simulink model "RobotControl"  (R2016a)
settings: Solver=FixedStepDiscrete  StartTime=0.0  StopTime=16  FixedStep=0.005  RelTol=1e-3
undefined symbols (not defined in the file or in its folder): CAL_EAST, CAL_NORTH, CAL_SOUTH, CAL_thetaGain, CAL_WEST, ENU_END, ENU_FORWARD, ENU_GTSP, ENU_LEFT_BUSY_RIGHT_BUSY, ENU_LEFT_BUSY_RIGHT_CLEANED, ENU_LEFT_BUSY_RIGHT_EMPTY, ENU_LEFT_CLEANED_RIGHT_BUSY, ENU_LEFT_CLEANED_RIGHT_CLEANED, ENU_LEFT_CLEANED_RIGHT_EMPTY, ENU_LEFT_EMPTY_RIGHT_BUSY, ENU_LEFT_EMPTY_RIGHT_CLEANED, ENU_LEFT_EMPTY_RIGHT_EMPTY, ENU_MOVE_TURN_LEFT, ENU_MOVE_TURN_RIGHT, ENU_MOVE_U_TURN, ENU_MOVE_U_TURN_LEFT, ENU_MOVE_U_TURN_RIGHT, ENU_STOP, ENU_ZIGZAG, ROTH, Routines
libraries: COMH x1, MOVH x1, SCAN x1, MOTH x1
settings Model: Creator=oelkawok  LastModifiedBy=oelkawok
settings DataIOCC: SaveOutput=off  SaveTime=off
settings DebuggingCC: AlgebraicLoopMsg=error  UnnecessaryDatatypeConvMsg=warning  SFcnCompatibilityMsg=warning

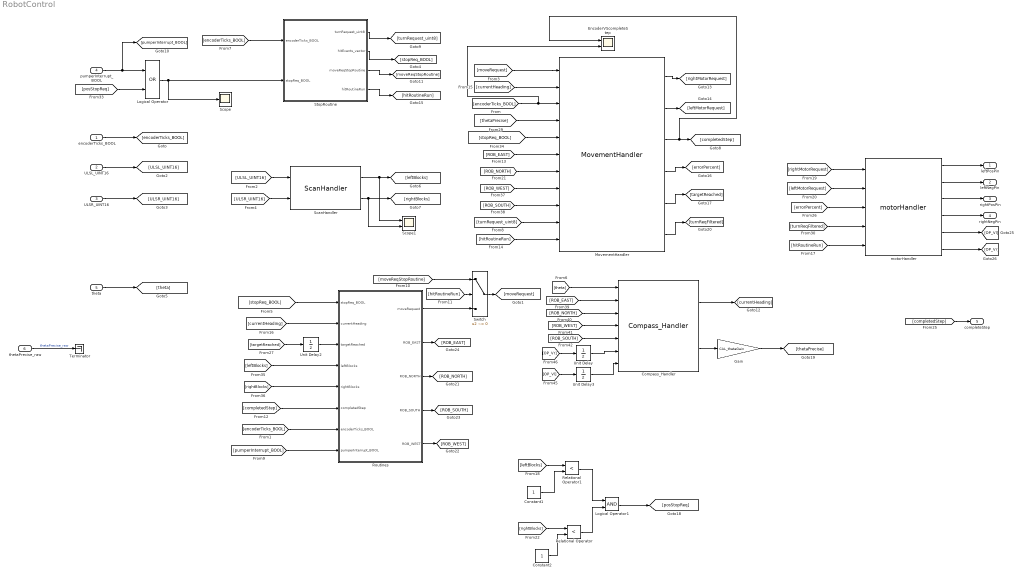
== system RobotControl ==
  encoderTicks_BOOL : Inport  OutDataTypeStr=boolean  PortDimensions=1
  ULSL_UINT16 : Inport  Port=2  PortDimensions=1
  ULSR_UINT16 : Inport  Port=3  PortDimensions=1
  pumperInterrupt_BOOL : Inport  Port=4  OutDataTypeStr=boolean  PortDimensions=1
  theta : Inport  Port=5  OutDataTypeStr=int16  PortDimensions=1
  thetaPrecise_raw : Inport  Port=6  OutDataTypeStr=uint16  PortDimensions=1
  Compass_Handler : COMH/Compass_Handler
  Constant1 : Constant
  Constant2 : Constant
  EncoderVScompleteStep : Scope  NumInputPorts=2
  Gain : Gain  Gain=CAL_thetaGain
  Logical Operator : Logic  Operator=OR  AllPortsSameDT=off  OutDataTypeStr=boolean
  Logical Operator1 : Logic  AllPortsSameDT=off  OutDataTypeStr=boolean
  MovementHandler : MOVH/MovementHandler
  Relational Operator : RelationalOperator  Operator=<  OutDataTypeStr=boolean
  Relational Operator1 : RelationalOperator  Operator=<  OutDataTypeStr=boolean
  Routines : Subsystem  AncestorBlock=ROTH/Routines
  ScanHandler : SCAN/ScanHandler
  Scope : Scope
  Scope1 : Scope  NumInputPorts=2
  StopRoutine : Subsystem
  Switch : Switch  Criteria=u2 ~= 0
  Terminator : Terminator
  Unit Delay : UnitDelay  SampleTime=-1
  Unit Delay2 : UnitDelay  SampleTime=-1
  Unit Delay3 : UnitDelay  SampleTime=-1
  motorHandler : MOTH/motorHandler
  leftPosPin : Outport  OutDataTypeStr=uint8  PortDimensions=1
  leftNegPin : Outport  Port=2  OutDataTypeStr=uint8  PortDimensions=1
  rightPosPin : Outport  Port=3  OutDataTypeStr=uint8  PortDimensions=1
  rightNegPin : Outport  Port=4  OutDataTypeStr=uint8  PortDimensions=1
  completeStep : Outport  Port=5  PortDimensions=1
  wires:
  [moveRequest] -> MovementHandler/1
  [encoderTicks_BOOL] -> EncoderVScompleteStep/2, MovementHandler/3
  encoderTicks_BOOL/1 -> [encoderTicks_BOOL]
  ULSL_UINT16/1 -> [ULSL_UINT16]
  [ULSL_UINT16] -> ScanHandler/1
  ULSR_UINT16/1 -> [ULSR_UINT16]
  [ULSR_UINT16] -> ScanHandler/2
  [theta] -> Compass_Handler/1
  ScanHandler/1 -> Scope1/1, [leftBlocks]
  ScanHandler/2 -> Scope1/2, [rightBlocks]
  MovementHandler/3 -> EncoderVScompleteStep/1, [completedStep]
  Compass_Handler/1 -> [currentHeading]
  [currentHeading] -> MovementHandler/2
  [rightMotorRequest] -> motorHandler/1
  [leftMotorRequest] -> motorHandler/2
  MovementHandler/2 -> [leftMotorRequest]
  MovementHandler/1 -> [rightMotorRequest]
  motorHandler/4 -> rightNegPin/1
  motorHandler/2 -> leftNegPin/1
  motorHandler/3 -> rightPosPin/1
  motorHandler/1 -> leftPosPin/1
  [completedStep] -> completeStep/1
  [errorPercent] -> motorHandler/3
  MovementHandler/4 -> [errorPercent]
  MovementHandler/5 -> [targetReached]
  [targetReached] -> Unit Delay2/1
  theta/1 -> [theta]
  [thetaPrecise] -> MovementHandler/4
  MovementHandler/6 -> [turnReqFiltered]
  [turnReqFiltered] -> motorHandler/4
  pumperInterrupt_BOOL/1 -> [pumperInterrupt_BOOL], Logical Operator/1
  [posStopReq] -> Logical Operator/2
  Logical Operator/1 -> Scope/1, StopRoutine/2(stopReq_BOOL)
  [stopReq_BOOL] -> MovementHandler/5
  Unit Delay2/1 -> Routines/3(targetReached)
  [stopReq_BOOL] -> Routines/1(stopReq_BOOL)
  [rightBlocks] -> Routines/5(rightBlocks)
  [leftBlocks] -> Routines/4(leftBlocks)
  [currentHeading] -> Routines/2(currentHeading)
  Logical Operator1/1 -> [posStopReq]
  [completedStep] -> Routines/6(completedStep)
  Routines/3(ROB_NORTH) -> [ROB_NORTH]
  Routines/2(ROB_EAST) -> [ROB_EAST]
  Routines/4(ROB_SOUTH) -> [ROB_SOUTH]
  Routines/5(ROB_WEST) -> [ROB_WEST]
  [ROB_NORTH] -> MovementHandler/7
  [ROB_EAST] -> MovementHandler/6
  [ROB_WEST] -> MovementHandler/8
  [ROB_SOUTH] -> MovementHandler/9
  [ROB_EAST] -> Compass_Handler/2
  [ROB_NORTH] -> Compass_Handler/3
  [ROB_WEST] -> Compass_Handler/4
  [ROB_SOUTH] -> Compass_Handler/5
  motorHandler/5 -> [OP_Vl]
  motorHandler/6 -> [OP_Vr]
  [OP_Vr] -> Unit Delay/1
  [OP_Vl] -> Unit Delay3/1
  Unit Delay/1 -> Compass_Handler/6
  Unit Delay3/1 -> Compass_Handler/7
  Compass_Handler/2 -> Gain/1
  Gain/1 -> [thetaPrecise]
  thetaPrecise_raw/1 -> Terminator/1  "thetaPrecise_raw"
  [encoderTicks_BOOL] -> Routines/7(encoderTicks_BOOL)
  [encoderTicks_BOOL] -> StopRoutine/1(encoderTicks_BOOL)
  StopRoutine/2(hitEvents_vector) -> [stopReq_BOOL]
  StopRoutine/1(turnRequest_uint8) -> [turnRequest_uint8]
  [turnRequest_uint8] -> MovementHandler/10
  [pumperInterrupt_BOOL] -> Routines/8(pumperInterrupt_BOOL)
  StopRoutine/3(moveReqStopRoutine) -> [moveReqStopRoutine]
  Switch/1 -> [moveRequest]
  Routines/1(moveRequest) -> Switch/3
  [moveReqStopRoutine] -> Switch/1
  StopRoutine/4(hitRoutineRun) -> [hitRoutineRun]
  [hitRoutineRun] -> Switch/2
  [hitRoutineRun] -> MovementHandler/11
  [hitRoutineRun] -> motorHandler/5
  [rightBlocks] -> Relational Operator/1
  Constant2/1 -> Relational Operator/2
  [leftBlocks] -> Relational Operator1/1
  Constant1/1 -> Relational Operator1/2
  Relational Operator1/1 -> Logical Operator1/1
  Relational Operator/1 -> Logical Operator1/2

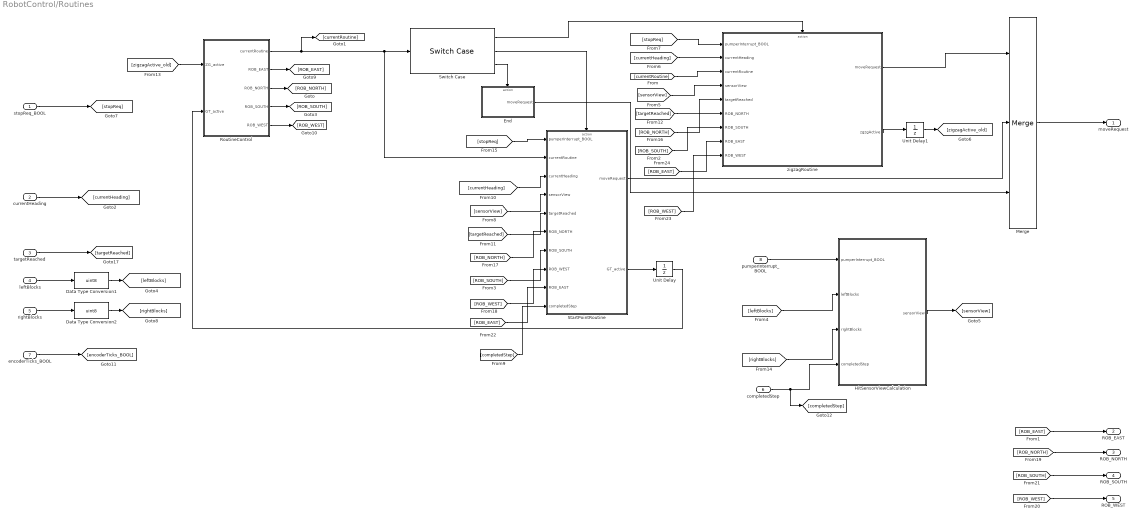
== system RobotControl/Routines ==
  stopReq_BOOL : Inport
  currentHeading : Inport  Port=2
  targetReached : Inport  Port=3
  leftBlocks : Inport  Port=4
  rightBlocks : Inport  Port=5
  completedStep : Inport  Port=6
  encoderTicks_BOOL : Inport  Port=7
  pumperInterrupt_BOOL : Inport  Port=8
  Data Type Conversion1 : DataTypeConversion  OutDataTypeStr=uint8
  Data Type Conversion2 : DataTypeConversion  OutDataTypeStr=uint8
  End : Subsystem  TreatAsAtomicUnit=on
  HitSensorViewCalculation : Subsystem
  Merge : Merge  Inputs=3  InitialOutput=5
      settings: AttributesFormatString=%<InitialOutput>
  RoutineControl : Subsystem
  StartPointRoutine : Subsystem
  Switch Case : SwitchCase  CaseConditions={ENU_ZIGZAG, ENU_GTSP, ENU_END}  ShowDefaultCase=off
      settings: AttributesFormatString=%<CaseConditions>
  Unit Delay : UnitDelay  InitialCondition=true  SampleTime=-1
      settings: AttributesFormatString=%<InitialCondition>
  Unit Delay1 : UnitDelay  InitialCondition=false  SampleTime=-1
      settings: AttributesFormatString=%<InitialCondition>
  zigzagRoutine : Subsystem
  moveRequest : Outport
  ROB_EAST : Outport  Port=2
  ROB_NORTH : Outport  Port=3
  ROB_SOUTH : Outport  Port=4
  ROB_WEST : Outport  Port=5
  wires:
  completedStep/1 -> [completedStep], HitSensorViewCalculation/4(completedStep)
  [leftBlocks] -> HitSensorViewCalculation/2(leftBlocks)
  [rightBlocks] -> HitSensorViewCalculation/3(rightBlocks)
  Data Type Conversion2/1 -> [rightBlocks]
  Data Type Conversion1/1 -> [leftBlocks]
  rightBlocks/1 -> Data Type Conversion2/1
  leftBlocks/1 -> Data Type Conversion1/1
  [zigzagActive_old] -> RoutineControl/1(ZG_active)
  Unit Delay1/1 -> [zigzagActive_old]
  [currentRoutine] -> zigzagRoutine/3(currentRoutine)
  currentHeading/1 -> [currentHeading]
  Unit Delay/1 -> RoutineControl/2(GT_active)
  StartPointRoutine/2(GT_active) -> Unit Delay/1
  Merge/1 -> moveRequest/1
  HitSensorViewCalculation/1(sensorView) -> [sensorView]
  [sensorView] -> zigzagRoutine/4(sensorView)
  [stopReq] -> zigzagRoutine/1(pumperInterrupt_BOOL)
  [currentHeading] -> zigzagRoutine/2(currentHeading)
  RoutineControl/1(currentRoutine) -> StartPointRoutine/2(currentRoutine), Switch Case/1, [currentRoutine]
  Switch Case/1 -> zigzagRoutine/Action
  Switch Case/2 -> StartPointRoutine/Action
  pumperInterrupt_BOOL/1 -> HitSensorViewCalculation/1(pumperInterrupt_BOOL)
  StartPointRoutine/1(moveRequest) -> Merge/2
  zigzagRoutine/1(moveRequest) -> Merge/1
  zigzagRoutine/2(zgzgActive) -> Unit Delay1/1
  [stopReq] -> StartPointRoutine/1(pumperInterrupt_BOOL)
  [sensorView] -> StartPointRoutine/4(sensorView)
  [currentHeading] -> StartPointRoutine/3(currentHeading)
  targetReached/1 -> [targetReached]
  [targetReached] -> StartPointRoutine/5(targetReached)
  [targetReached] -> zigzagRoutine/5(targetReached)
  stopReq_BOOL/1 -> [stopReq]
  RoutineControl/3(ROB_NORTH) -> [ROB_NORTH]
  RoutineControl/2(ROB_EAST) -> [ROB_EAST]
  RoutineControl/5(ROB_WEST) -> [ROB_WEST]
  RoutineControl/4(ROB_SOUTH) -> [ROB_SOUTH]
  [ROB_SOUTH] -> zigzagRoutine/7(ROB_SOUTH)
  [ROB_SOUTH] -> StartPointRoutine/7(ROB_SOUTH)
  [ROB_NORTH] -> zigzagRoutine/6(ROB_NORTH)
  [ROB_NORTH] -> StartPointRoutine/6(ROB_NORTH)
  [ROB_WEST] -> StartPointRoutine/8(ROB_WEST)
  [ROB_EAST] -> ROB_EAST/1
  [ROB_NORTH] -> ROB_NORTH/1
  [ROB_SOUTH] -> ROB_SOUTH/1
  [ROB_WEST] -> ROB_WEST/1
  [ROB_EAST] -> StartPointRoutine/9(ROB_EAST)
  Switch Case/3 -> End/Action
  End/1(moveRequest) -> Merge/3
  encoderTicks_BOOL/1 -> [encoderTicks_BOOL]
  [completedStep] -> StartPointRoutine/10(completedStep)
  [ROB_EAST] -> zigzagRoutine/8(ROB_EAST)
  [ROB_WEST] -> zigzagRoutine/9(ROB_WEST)

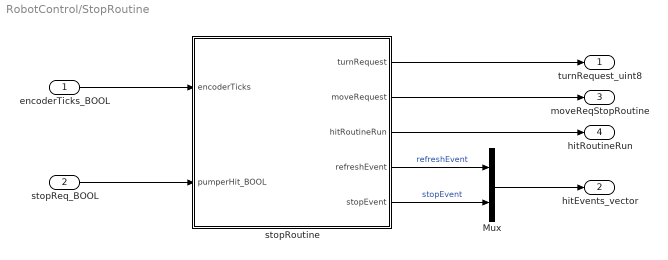
== system RobotControl/StopRoutine ==
  encoderTicks_BOOL : Inport
  stopReq_BOOL : Inport  Port=2
  Mux : Mux  Inputs=2
  stopRoutine : Stateflow chart  TreatAsAtomicUnit=on
  turnRequest_uint8 : Outport
  hitEvents_vector : Outport  Port=2
  moveReqStopRoutine : Outport  Port=3
  hitRoutineRun : Outport  Port=4
  wires:
  stopRoutine/5(stopEvent) -> Mux/2  "stopEvent"
  stopRoutine/1(turnRequest) -> turnRequest_uint8/1
  stopReq_BOOL/1 -> stopRoutine/2(pumperHit_BOOL)
  encoderTicks_BOOL/1 -> stopRoutine/1(encoderTicks)
  stopRoutine/4(refreshEvent) -> Mux/1  "refreshEvent"
  Mux/1 -> hitEvents_vector/1
  stopRoutine/2(moveRequest) -> moveReqStopRoutine/1
  stopRoutine/3(hitRoutineRun) -> hitRoutineRun/1

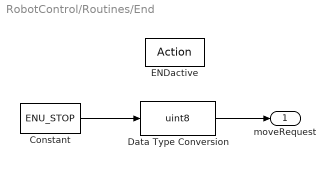
== system RobotControl/Routines/End ==
  ENDactive : ActionPort  ActionType=case
  Constant : Constant  Value=ENU_STOP
  Data Type Conversion : DataTypeConversion  OutDataTypeStr=uint8
  moveRequest : Outport
  wires:
  Constant/1 -> Data Type Conversion/1
  Data Type Conversion/1 -> moveRequest/1

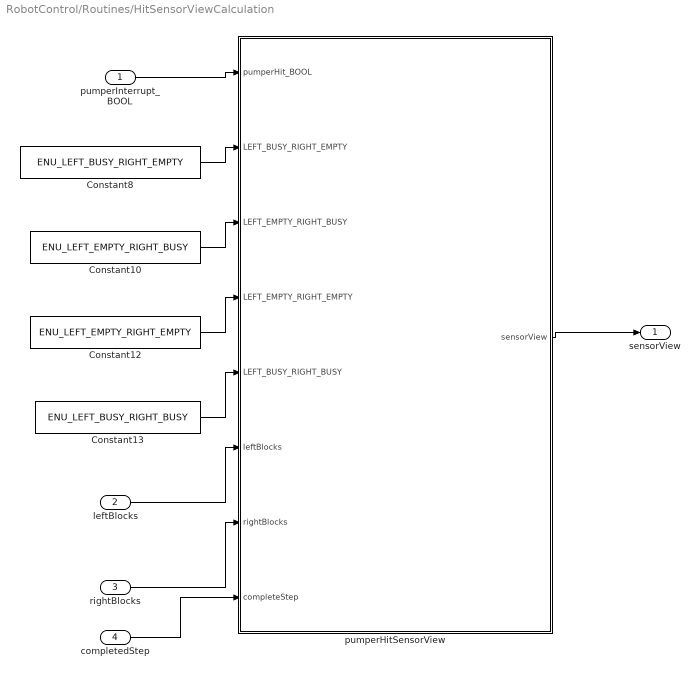
== system RobotControl/Routines/HitSensorViewCalculation ==
  pumperInterrupt_BOOL : Inport
  leftBlocks : Inport  Port=2
  rightBlocks : Inport  Port=3
  completedStep : Inport  Port=4
  Constant10 : Constant  Value=ENU_LEFT_EMPTY_RIGHT_BUSY
  Constant12 : Constant  Value=ENU_LEFT_EMPTY_RIGHT_EMPTY
  Constant13 : Constant  Value=ENU_LEFT_BUSY_RIGHT_BUSY
  Constant8 : Constant  Value=ENU_LEFT_BUSY_RIGHT_EMPTY
  pumperHitSensorView : Stateflow chart  TreatAsAtomicUnit=on
  sensorView : Outport
  wires:
  completedStep/1 -> pumperHitSensorView/8(completeStep)
  rightBlocks/1 -> pumperHitSensorView/7(rightBlocks)
  leftBlocks/1 -> pumperHitSensorView/6(leftBlocks)
  pumperHitSensorView/1(sensorView) -> sensorView/1
  Constant13/1 -> pumperHitSensorView/5(LEFT_BUSY_RIGHT_BUSY)
  Constant12/1 -> pumperHitSensorView/4(LEFT_EMPTY_RIGHT_EMPTY)
  Constant10/1 -> pumperHitSensorView/3(LEFT_EMPTY_RIGHT_BUSY)
  Constant8/1 -> pumperHitSensorView/2(LEFT_BUSY_RIGHT_EMPTY)
  pumperInterrupt_BOOL/1 -> pumperHitSensorView/1(pumperHit_BOOL)

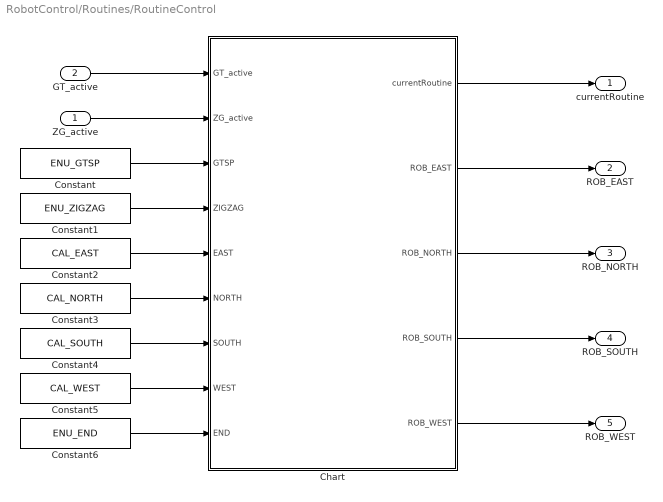
== system RobotControl/Routines/RoutineControl ==
  ZG_active : Inport
  GT_active : Inport  Port=2
  Chart : Stateflow chart  TreatAsAtomicUnit=on
  Constant : Constant  Value=ENU_GTSP
  Constant1 : Constant  Value=ENU_ZIGZAG
  Constant2 : Constant  Value=CAL_EAST
  Constant3 : Constant  Value=CAL_NORTH
  Constant4 : Constant  Value=CAL_SOUTH
  Constant5 : Constant  Value=CAL_WEST
  Constant6 : Constant  Value=ENU_END
  currentRoutine : Outport
  ROB_EAST : Outport  Port=2
  ROB_NORTH : Outport  Port=3
  ROB_SOUTH : Outport  Port=4
  ROB_WEST : Outport  Port=5
  wires:
  Constant1/1 -> Chart/4(ZIGZAG)
  Constant/1 -> Chart/3(GTSP)
  Chart/1(currentRoutine) -> currentRoutine/1
  GT_active/1 -> Chart/1(GT_active)
  ZG_active/1 -> Chart/2(ZG_active)
  Constant2/1 -> Chart/5(EAST)
  Constant5/1 -> Chart/8(WEST)
  Constant3/1 -> Chart/6(NORTH)
  Constant4/1 -> Chart/7(SOUTH)
  Chart/2(ROB_EAST) -> ROB_EAST/1
  Chart/3(ROB_NORTH) -> ROB_NORTH/1
  Chart/4(ROB_SOUTH) -> ROB_SOUTH/1
  Chart/5(ROB_WEST) -> ROB_WEST/1
  Constant6/1 -> Chart/9(END)

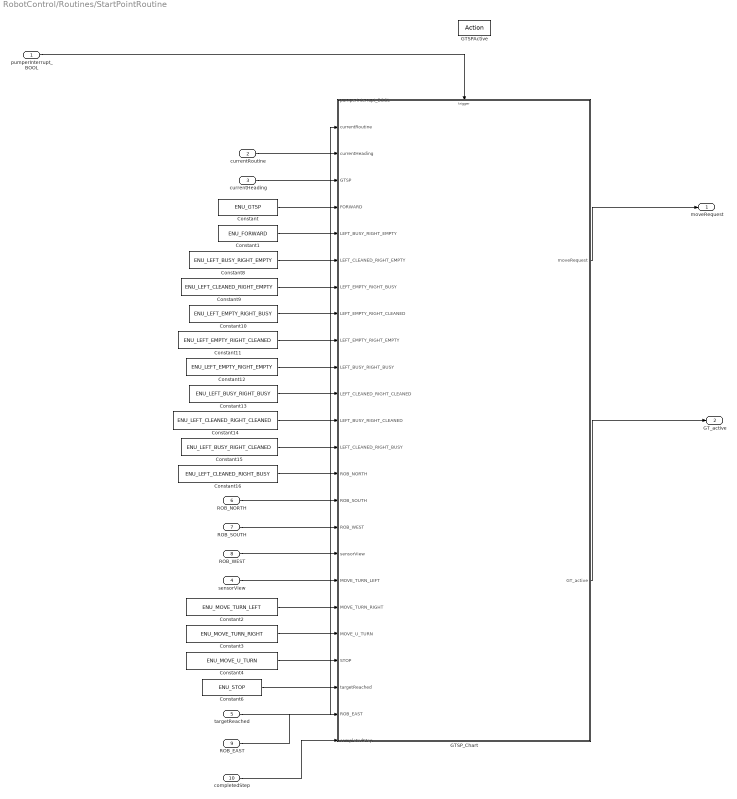
== system RobotControl/Routines/StartPointRoutine ==
  pumperInterrupt_BOOL : Inport
  currentRoutine : Inport  Port=2
  currentHeading : Inport  Port=3
  sensorView : Inport  Port=4
  targetReached : Inport  Port=5
  ROB_NORTH : Inport  Port=6
  ROB_SOUTH : Inport  Port=7
  ROB_WEST : Inport  Port=8
  ROB_EAST : Inport  Port=9
  completedStep : Inport  Port=10
  GTSPActive : ActionPort  ActionType=case
  Constant : Constant  Value=ENU_GTSP
  Constant1 : Constant  Value=ENU_FORWARD
  Constant10 : Constant  Value=ENU_LEFT_EMPTY_RIGHT_BUSY
  Constant11 : Constant  Value=ENU_LEFT_EMPTY_RIGHT_CLEANED
  Constant12 : Constant  Value=ENU_LEFT_EMPTY_RIGHT_EMPTY
  Constant13 : Constant  Value=ENU_LEFT_BUSY_RIGHT_BUSY
  Constant14 : Constant  Value=ENU_LEFT_CLEANED_RIGHT_CLEANED
  Constant15 : Constant  Value=ENU_LEFT_BUSY_RIGHT_CLEANED
  Constant16 : Constant  Value=ENU_LEFT_CLEANED_RIGHT_BUSY
  Constant2 : Constant  Value=ENU_MOVE_TURN_LEFT
  Constant3 : Constant  Value=ENU_MOVE_TURN_RIGHT
  Constant4 : Constant  Value=ENU_MOVE_U_TURN
  Constant6 : Constant  Value=ENU_STOP
  Constant8 : Constant  Value=ENU_LEFT_BUSY_RIGHT_EMPTY
  Constant9 : Constant  Value=ENU_LEFT_CLEANED_RIGHT_EMPTY
  GTSP_Chart : Stateflow chart  TreatAsAtomicUnit=on
  moveRequest : Outport
  GT_active : Outport  Port=2
  wires:
  Constant6/1 -> GTSP_Chart/22(STOP)
  GTSP_Chart/2(GT_active) -> GT_active/1
  Constant2/1 -> GTSP_Chart/19(MOVE_TURN_LEFT)
  Constant3/1 -> GTSP_Chart/20(MOVE_TURN_RIGHT)
  Constant4/1 -> GTSP_Chart/21(MOVE_U_TURN)
  sensorView/1 -> GTSP_Chart/18(sensorView)
  ROB_NORTH/1 -> GTSP_Chart/15(ROB_NORTH)
  ROB_SOUTH/1 -> GTSP_Chart/16(ROB_SOUTH)
  ROB_WEST/1 -> GTSP_Chart/17(ROB_WEST)
  Constant16/1 -> GTSP_Chart/14(LEFT_CLEANED_RIGHT_BUSY)
  Constant15/1 -> GTSP_Chart/13(LEFT_BUSY_RIGHT_CLEANED)
  Constant14/1 -> GTSP_Chart/12(LEFT_CLEANED_RIGHT_CLEANED)
  Constant13/1 -> GTSP_Chart/11(LEFT_BUSY_RIGHT_BUSY)
  Constant12/1 -> GTSP_Chart/10(LEFT_EMPTY_RIGHT_EMPTY)
  Constant11/1 -> GTSP_Chart/9(LEFT_EMPTY_RIGHT_CLEANED)
  Constant10/1 -> GTSP_Chart/8(LEFT_EMPTY_RIGHT_BUSY)
  Constant9/1 -> GTSP_Chart/7(LEFT_CLEANED_RIGHT_EMPTY)
  Constant8/1 -> GTSP_Chart/6(LEFT_BUSY_RIGHT_EMPTY)
  Constant1/1 -> GTSP_Chart/5(FORWARD)
  Constant/1 -> GTSP_Chart/4(GTSP)
  currentRoutine/1 -> GTSP_Chart/2(currentRoutine)
  currentHeading/1 -> GTSP_Chart/3(currentHeading)
  targetReached/1 -> GTSP_Chart/23(targetReached)
  ROB_EAST/1 -> GTSP_Chart/24(ROB_EAST)
  GTSP_Chart/1(moveRequest) -> moveRequest/1
  pumperInterrupt_BOOL/1 -> GTSP_Chart/Trigger
  completedStep/1 -> GTSP_Chart/25(completedStep)

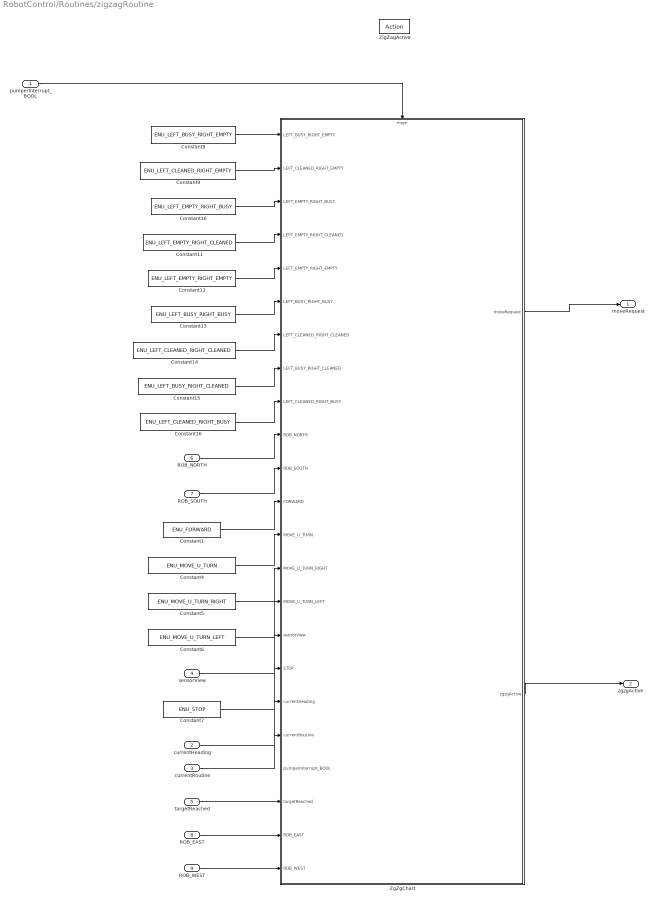
== system RobotControl/Routines/zigzagRoutine ==
  pumperInterrupt_BOOL : Inport
  currentHeading : Inport  Port=2
  currentRoutine : Inport  Port=3
  sensorView : Inport  Port=4
  targetReached : Inport  Port=5
  ROB_NORTH : Inport  Port=6
  ROB_SOUTH : Inport  Port=7
  ROB_EAST : Inport  Port=8
  ROB_WEST : Inport  Port=9
  ZigZagActive : ActionPort  ActionType=case
  Constant1 : Constant  Value=ENU_FORWARD
  Constant10 : Constant  Value=ENU_LEFT_EMPTY_RIGHT_BUSY
  Constant11 : Constant  Value=ENU_LEFT_EMPTY_RIGHT_CLEANED
  Constant12 : Constant  Value=ENU_LEFT_EMPTY_RIGHT_EMPTY
  Constant13 : Constant  Value=ENU_LEFT_BUSY_RIGHT_BUSY
  Constant14 : Constant  Value=ENU_LEFT_CLEANED_RIGHT_CLEANED
  Constant15 : Constant  Value=ENU_LEFT_BUSY_RIGHT_CLEANED
  Constant16 : Constant  Value=ENU_LEFT_CLEANED_RIGHT_BUSY
  Constant4 : Constant  Value=ENU_MOVE_U_TURN
  Constant5 : Constant  Value=ENU_MOVE_U_TURN_RIGHT
  Constant6 : Constant  Value=ENU_MOVE_U_TURN_LEFT
  Constant7 : Constant  Value=ENU_STOP
  Constant8 : Constant  Value=ENU_LEFT_BUSY_RIGHT_EMPTY
  Constant9 : Constant  Value=ENU_LEFT_CLEANED_RIGHT_EMPTY
  ZgZgChart : Stateflow chart  TreatAsAtomicUnit=on
  moveRequest : Outport
  zgzgActive : Outport  Port=2  InitialOutput=true
  wires:
  Constant8/1 -> ZgZgChart/1(LEFT_BUSY_RIGHT_EMPTY)
  Constant9/1 -> ZgZgChart/2(LEFT_CLEANED_RIGHT_EMPTY)
  Constant13/1 -> ZgZgChart/6(LEFT_BUSY_RIGHT_BUSY)
  Constant15/1 -> ZgZgChart/8(LEFT_BUSY_RIGHT_CLEANED)
  ROB_NORTH/1 -> ZgZgChart/10(ROB_NORTH)
  ROB_SOUTH/1 -> ZgZgChart/11(ROB_SOUTH)
  Constant14/1 -> ZgZgChart/7(LEFT_CLEANED_RIGHT_CLEANED)
  Constant11/1 -> ZgZgChart/4(LEFT_EMPTY_RIGHT_CLEANED)
  Constant12/1 -> ZgZgChart/5(LEFT_EMPTY_RIGHT_EMPTY)
  Constant10/1 -> ZgZgChart/3(LEFT_EMPTY_RIGHT_BUSY)
  Constant16/1 -> ZgZgChart/9(LEFT_CLEANED_RIGHT_BUSY)
  Constant1/1 -> ZgZgChart/12(FORWARD)
  Constant4/1 -> ZgZgChart/13(MOVE_U_TURN)
  Constant6/1 -> ZgZgChart/15(MOVE_U_TURN_LEFT)
  Constant5/1 -> ZgZgChart/14(MOVE_U_TURN_RIGHT)
  sensorView/1 -> ZgZgChart/16(sensorView)
  currentRoutine/1 -> ZgZgChart/19(currentRoutine)
  currentHeading/1 -> ZgZgChart/18(currentHeading)
  Constant7/1 -> ZgZgChart/17(STOP)
  ZgZgChart/2(zgzgActive) -> zgzgActive/1
  targetReached/1 -> ZgZgChart/21(targetReached)
  ZgZgChart/1(moveRequest) -> moveRequest/1
  pumperInterrupt_BOOL/1 -> ZgZgChart/Trigger
  ROB_WEST/1 -> ZgZgChart/23(ROB_WEST)
  ROB_EAST/1 -> ZgZgChart/22(ROB_EAST)

== stateflow chart RobotControl/Routines/StartPointRoutine/GTSP_Chart ==
  state Idle
    entry:
    counter = 0;
    moveRequest = STOP;
    step1Flag = false;
    GT_active = true;
    du:
    counter++;
  state GTSP_Active
    state Forward
      entry:
      moveRequest = FORWARD;
    state TurnLeft
      entry:
      moveRequest = MOVE_TURN_LEFT;
    state preFinishLeftBlockedN
      entry:
      moveRequest = MOVE_U_TURN;
    state preFinishLeftBlockedW
      entry:
      moveRequest = MOVE_TURN_RIGHT;
    state preFinishNormal
      entry:
      moveRequest = MOVE_TURN_LEFT;
    state preFinishBlockedW
    state preFinishBlockedN
      entry:
      moveRequest = MOVE_U_TURN;
    state finishedGTSP
      entry:
      step1Flag = true;
      moveRequest = STOP;
    TurnLeft -> Forward : [(currentHeading == ROB_WEST)...
        | && (targetReached == true)]
    (default) -> Forward
    Forward -> (junction 14) : stopEvent
    (junction 14) -> (junction 17) [order 1] : [(sensorView == LEFT_EMPTY_RIGHT_EMPTY)...
        | || (sensorView == LEFT_EMPTY_RIGHT_CLEANED)...
        | || (sensorView == LEFT_EMPTY_RIGHT_BUSY)]
    (junction 14) -> (junction 22) [order 2] : [(sensorView == LEFT_CLEANED_RIGHT_EMPTY)...
        | || (sensorView == LEFT_BUSY_RIGHT_EMPTY)]
    (junction 14) -> (junction 29) [order 3] : [(sensorView == LEFT_BUSY_RIGHT_BUSY)...
        | || (sensorView == LEFT_BUSY_RIGHT_CLEANED)...
        | || (sensorView == LEFT_CLEANED_RIGHT_BUSY)...
        | || (sensorView == LEFT_CLEANED_RIGHT_CLEANED)]
    (junction 17) -> TurnLeft [order 1] : [currentHeading == ROB_NORTH]
    (junction 17) -> preFinishNormal [order 2] : [currentHeading == ROB_WEST]
    (junction 22) -> preFinishLeftBlockedW [order 2] : [currentHeading == ROB_WEST]
    (junction 22) -> preFinishLeftBlockedN [order 1] : [currentHeading == ROB_NORTH]
    (junction 29) -> preFinishBlockedW [order 1] : [currentHeading == ROB_WEST]
    (junction 29) -> preFinishBlockedN [order 2] : [currentHeading == ROB_NORTH]
    preFinishLeftBlockedW -> finishedGTSP : [(currentHeading == ROB_NORTH)...
        | && (targetReached == true)]
    preFinishNormal -> finishedGTSP : [(currentHeading == ROB_SOUTH)...
        | && (targetReached == true)]
    preFinishBlockedN -> finishedGTSP : [(currentHeading == ROB_NORTH)...
        | && (targetReached == true)]
    preFinishBlockedW -> finishedGTSP
  state faceWest
    state turingRight
      entry:
      moveRequest = MOVE_U_TURN;
    state Start
      en:
      initHeading = false;
    state turningLeft
      entry:
      moveRequest = MOVE_TURN_RIGHT;
    state finishInit
      en:
      initHeading = true;
    state uturn
      entry:
      moveRequest = MOVE_TURN_LEFT;
    Start -> turingRight [order 1] : [currentHeading == ROB_SOUTH]
    turingRight -> (junction 135)
    (default) -> Start
    Start -> turningLeft [order 2] : [currentHeading == ROB_WEST]
    Start -> uturn [order 3] : [currentHeading == ROB_EAST]
    turningLeft -> (junction 135)
    (junction 135) -> finishInit : [currentHeading == ROB_NORTH]
    Start -> finishInit [order 4] : [currentHeading == ROB_NORTH]
    uturn -> (junction 135)
  state MostSouthLeft
    state start
    state facingNorth
      state GTSPsearch
        en:
        round = 0;
        state start
          en:
          moveRequest = FORWARD;
          round++;
        state furtherDown
          en:
          moveRequest = MOVE_TURN_LEFT;
        state countingGap
          entry:
          gapCounter = 0;
          du:
          gapCounter++;
        state emptyOnRight
          en:
          moveRequest = MOVE_TURN_RIGHT;
        state facingWest
          en:
          moveRequest = FORWARD;
        (default) -> MostSouthLeft.facingNorth.GTSPsearch.start
        MostSouthLeft.facingNorth.GTSPsearch.start -> MostSouthLeft.facingNorth.GTSPsearch.countingGap [order 2] : [sensorView == LEFT_BUSY_RIGHT_EMPTY...
            | || sensorView == LEFT_EMPTY_RIGHT_EMPTY]
        MostSouthLeft.facingNorth.GTSPsearch.furtherDown -> MostSouthLeft.facingNorth.GTSPsearch.start : [(currentHeading == ROB_SOUTH)...
            | && (targetReached)]
        (junction 123) -> MostSouthLeft.facingNorth.GTSPsearch.furtherDown [order 2] : [(sensorView == LEFT_EMPTY_RIGHT_BUSY)...
            | || (sensorView == LEFT_EMPTY_RIGHT_EMPTY)]
        MostSouthLeft.facingNorth.GTSPsearch.countingGap -> MostSouthLeft.facingNorth.GTSPsearch.emptyOnRight : [(sensorView == LEFT_BUSY_RIGHT_EMPTY...
            | || sensorView == LEFT_EMPTY_RIGHT_EMPTY) ...
            | && (gapCounter >= 100)]
        MostSouthLeft.facingNorth.GTSPsearch.facingWest -> (junction 123) : [pumperInterrupt_BOOL]
            | /moveRequest = STOP;
        MostSouthLeft.facingNorth.GTSPsearch.emptyOnRight -> MostSouthLeft.facingNorth.GTSPsearch.facingWest : [(currentHeading == ROB_WEST)...
            | && (targetReached)]
      state End
        en:
        activeFlag = false;
      (default) -> MostSouthLeft.facingNorth.GTSPsearch
      MostSouthLeft.facingNorth.GTSPsearch -> MostSouthLeft.facingNorth.End : [(currentHeading == ROB_SOUTH)...
          | && (targetReached)...
          | && (pumperInterrupt_BOOL)...
          | && (round > 1)]
          | /moveRequest = STOP;
      MostSouthLeft.facingNorth.GTSPsearch.start -> MostSouthLeft.facingNorth.End [order 1] : [pumperInterrupt_BOOL]
          | /moveRequest = STOP;
      (junction 123) -> MostSouthLeft.facingNorth.End [order 1] : [(sensorView == LEFT_BUSY_RIGHT_BUSY)...
          | || (sensorView == LEFT_BUSY_RIGHT_EMPTY)]
    state finish
      en:
      GT_active = false;
    state facingSouth
      state GTSPsearch
        en:
        round = 0;
        state start
          en:
          moveRequest = FORWARD;
          round++;
        state furtherDown
          en:
          moveRequest = MOVE_TURN_LEFT;
        state countingGap
          entry:
          gapCounter = 0;
          du:
          gapCounter++;
        state emptyOnRight
          en:
          moveRequest = MOVE_TURN_RIGHT;
        state facingWest
          en:
          moveRequest = FORWARD;
        (default) -> MostSouthLeft.facingSouth.GTSPsearch.start
        MostSouthLeft.facingSouth.GTSPsearch.furtherDown -> MostSouthLeft.facingSouth.GTSPsearch.start : [(currentHeading == ROB_SOUTH)...
            | && (targetReached)]
        MostSouthLeft.facingSouth.GTSPsearch.start -> MostSouthLeft.facingSouth.GTSPsearch.emptyOnRight [order 2] : [hasChanged(completedStep) ...
            | && (sensorView == LEFT_BUSY_RIGHT_EMPTY...
            | || sensorView == LEFT_EMPTY_RIGHT_EMPTY)]
        MostSouthLeft.facingSouth.GTSPsearch.start -> (junction 162) [order 1] : stopEvent
        (junction 88) -> MostSouthLeft.facingSouth.GTSPsearch.furtherDown [order 2] : [(sensorView == LEFT_EMPTY_RIGHT_BUSY)...
            | || (sensorView == LEFT_EMPTY_RIGHT_EMPTY)]
        (junction 162) -> MostSouthLeft.facingSouth.GTSPsearch.emptyOnRight : [(sensorView == LEFT_BUSY_RIGHT_EMPTY...
            | || sensorView == LEFT_EMPTY_RIGHT_EMPTY)]
        MostSouthLeft.facingSouth.GTSPsearch.countingGap -> MostSouthLeft.facingSouth.GTSPsearch.emptyOnRight : [(sensorView == LEFT_BUSY_RIGHT_EMPTY...
            | || sensorView == LEFT_EMPTY_RIGHT_EMPTY) ...
            | && (gapCounter >= CAL_GTSPgapCounter)]
        MostSouthLeft.facingSouth.GTSPsearch.facingWest -> (junction 88) : stopEvent
        MostSouthLeft.facingSouth.GTSPsearch.emptyOnRight -> MostSouthLeft.facingSouth.GTSPsearch.facingWest : [(currentHeading == ROB_WEST)...
            | && (targetReached)]
      state End
        en:
        activeFlag = false;
      note: 
      (default) -> MostSouthLeft.facingSouth.GTSPsearch
      MostSouthLeft.facingSouth.GTSPsearch -> (junction 154) : stopEvent
      (junction 154) -> MostSouthLeft.facingSouth.End : [(currentHeading == ROB_SOUTH)...
          | && (targetReached)...
          | && (round > 1)]
          | /moveRequest = STOP;
      MostSouthLeft.facingSouth.GTSPsearch.start -> MostSouthLeft.facingSouth.End [order 3] : stopEvent
      (junction 88) -> MostSouthLeft.facingSouth.End [order 1] : [(sensorView == LEFT_BUSY_RIGHT_BUSY)...
          | || (sensorView == LEFT_BUSY_RIGHT_EMPTY)]
    (default) -> MostSouthLeft.start
    MostSouthLeft.start -> finish [order 2] : [currentHeading == ROB_NORTH]
    MostSouthLeft.start -> facingSouth [order 1] : [currentHeading == ROB_SOUTH]
    facingNorth -> finish : [activeFlag == false]
    facingSouth -> finish : [activeFlag == false]
  (default) -> Idle
  Idle -> faceWest : [(currentRoutine == GTSP)...
      | && (counter > CAL_GTSPdelayStart)]
  faceWest -> GTSP_Active : [initHeading == true]
  finish -> Idle : [currentRoutine == GTSP]
  GTSP_Active -> Idle [order 1] : [currentRoutine != GTSP]
  GTSP_Active -> MostSouthLeft [order 2] : [step1Flag == true]
      | /activeFlag = true;
  preFinishLeftBlockedN -> (junction 156) : [(currentHeading == ROB_SOUTH)...
      | && (targetReached == true)]
  (junction 156) -> finish
  data: pumperInterrupt_BOOL input; currentRoutine input; currentHeading input; GTSP input; FORWARD input; LEFT_BUSY_RIGHT_EMPTY input; LEFT_CLEANED_RIGHT_EMPTY input; LEFT_EMPTY_RIGHT_BUSY input; LEFT_EMPTY_RIGHT_CLEANED input; LEFT_EMPTY_RIGHT_EMPTY input; LEFT_BUSY_RIGHT_BUSY input; LEFT_CLEANED_RIGHT_CLEANED input; LEFT_BUSY_RIGHT_CLEANED input; LEFT_CLEANED_RIGHT_BUSY input; ROB_NORTH input; ROB_SOUTH input; ROB_WEST input; sensorView input; moveRequest output uint8; MOVE_TURN_LEFT input; MOVE_TURN_RIGHT input; MOVE_U_TURN input; GT_active output boolean =true; STOP input; targetReached input; counter local uint8; gapCounter local uint8; round local uint8; step1Flag local uint8; initHeading local boolean; ROB_EAST input; activeFlag local boolean; CAL_GTSPdelayStart constant uint8 =CAL_GTSPdelayStart; CAL_GTSPgapCounter constant uint8 =CAL_GTSPgapCounter; completedStep input
  events: refreshEvent input EITHER_EDGE_EVENT; stopEvent input EITHER_EDGE_EVENT

== stateflow chart RobotControl/Routines/HitSensorViewCalculation/pumperHitSensorView ==
  (default) -> (junction 68) : {
      | //sensorView = 0;
      | }
  (junction 68) -> (junction 69) [order 1] : [pumperHit_BOOL || completeStep]
  (junction 69) -> (junction 71)
  (junction 68) -> (junction 95) [order 2]
  (junction 71) -> (junction 73) [order 1] : [(leftBlocks <= 1) ...
      | && (rightBlocks >= 1)]
  (junction 71) -> (junction 101) [order 2]
  (junction 73) -> (junction 100) : {
      | sensorView = LEFT_BUSY_RIGHT_EMPTY;
      | }
  (junction 100) -> (junction 101)
  (junction 101) -> (junction 76)
  (junction 76) -> (junction 75) [order 1] : [(leftBlocks >= 1)...
      | && (rightBlocks <= 1)]
  (junction 76) -> (junction 102) [order 2]
  (junction 75) -> (junction 103) : {
      | sensorView = LEFT_EMPTY_RIGHT_BUSY;
      | }
  (junction 103) -> (junction 102)
  (junction 102) -> (junction 78)
  (junction 78) -> (junction 77) [order 1] : [(leftBlocks >= 1)...
      | && (rightBlocks >= 1)]
  (junction 78) -> (junction 104) [order 2]
  (junction 77) -> (junction 105) : {
      | sensorView = LEFT_EMPTY_RIGHT_EMPTY;
      | }
  (junction 105) -> (junction 104)
  (junction 104) -> (junction 80)
  (junction 80) -> (junction 79) [order 1] : [(leftBlocks < 1) ...
      | && (rightBlocks < 1)]
  (junction 80) -> (junction 91) [order 2]
  (junction 79) -> (junction 90) : {
      | sensorView = LEFT_BUSY_RIGHT_BUSY;
      | }
  (junction 91) -> (junction 95)
  (junction 90) -> (junction 91)
  (junction 95) -> (junction 98)
  data: pumperHit_BOOL input; sensorView output uint8; LEFT_BUSY_RIGHT_EMPTY input; LEFT_EMPTY_RIGHT_BUSY input; LEFT_EMPTY_RIGHT_EMPTY input; LEFT_BUSY_RIGHT_BUSY input; leftBlocks input; rightBlocks input; completeStep input

== stateflow chart RobotControl/Routines/RoutineControl/Chart ==
  state GTSP
    entry:
    currentRoutine = GTSP;
  state init
    en:
    zgzgCounter = 0;
  state ZIGZAG
    entry:
    currentRoutine = ZIGZAG;
    zgzgCounter++;
  state End
    en:
    currentRoutine = END;
  (default) -> init
  GTSP -> ZIGZAG : [(GT_active == false) && after(5,tick)]
  init -> GTSP : /ROB_NORTH = NORTH;
      | ROB_SOUTH = SOUTH;
      | ROB_WEST = WEST;
      | ROB_EAST = EAST;
  ZIGZAG -> GTSP [order 2] : [(ZG_active == false)...
      | && after(5, tick)]
      | /ROB_NORTH = WEST;
      | ROB_SOUTH = EAST;
      | ROB_WEST = SOUTH;
      | ROB_EAST = NORTH;
  ZIGZAG -> End [order 1] : [(ZG_active == false)...
      | && (zgzgCounter >= 2)...
      | && after(5 ,tick)]
  data: currentRoutine output uint8; GT_active input; ZG_active input; GTSP input; ZIGZAG input; zgzgCounter local uint8; ROB_EAST output uint16; ROB_NORTH output uint16; ROB_SOUTH output uint16; ROB_WEST output uint16; EAST input; NORTH input; SOUTH input; WEST input; END input

== stateflow chart RobotControl/Routines/zigzagRoutine/ZgZgChart ==
  state SwitchLane
  state finishZigZag
    en:
    zgzgActive = false;
    moveRequest = STOP;
  state MovingForward
    en:
    moveRequest = FORWARD;
  state Idle
    en:
    zgzgActive = true;
    finishCounter = 1;
  state faceWest
    state turingRight
      entry:
      moveRequest = MOVE_U_TURN;
    state Start
      en:
      initHeading = false;
    state turningLeft
      entry:
      moveRequest = MOVE_TURN_RIGHT;
    state finishInit
      en:
      initHeading = true;
    state uturn
      entry:
      moveRequest = MOVE_TURN_LEFT;
    Start -> turingRight [order 1] : [currentHeading == ROB_SOUTH]
    turingRight -> (junction 93)
    (default) -> Start
    Start -> turningLeft [order 2] : [currentHeading == ROB_WEST]
    Start -> uturn [order 3] : [currentHeading == ROB_EAST]
    turningLeft -> (junction 93)
    (junction 93) -> finishInit : [currentHeading == ROB_NORTH]
    Start -> finishInit [order 4] : [currentHeading == ROB_NORTH]
    uturn -> (junction 93)
  (junction 34) -> SwitchLane [order 1] : [currentHeading == ROB_NORTH]
      | /moveRequest = MOVE_U_TURN_RIGHT;
      | headingRequest = ROB_SOUTH;
      | finishCounter = 1;
  (junction 34) -> SwitchLane [order 2] : [currentHeading == ROB_SOUTH]
      | /moveRequest = MOVE_U_TURN_LEFT;
      | headingRequest = ROB_NORTH;
      | finishCounter = 1;
  (junction 35) -> SwitchLane [order 1] : [currentHeading == ROB_NORTH]
      | /moveRequest = MOVE_U_TURN_RIGHT;
      | headingRequest = ROB_SOUTH;
      | finishCounter = 1;
  (junction 33) -> (junction 34) [order 1] : [sensorView == LEFT_EMPTY_RIGHT_EMPTY]
  SwitchLane -> finishZigZag [order 1] : [finishCounter > CAL_ZgZgCounterThd]
  (junction 35) -> SwitchLane [order 2] : [currentHeading == ROB_SOUTH]
      | /moveRequest = MOVE_U_TURN;
      | headingRequest = ROB_NORTH;
      | finishCounter++;
  (junction 33) -> (junction 35) [order 2] : [(sensorView == LEFT_CLEANED_RIGHT_EMPTY)...
      | || (sensorView == LEFT_BUSY_RIGHT_EMPTY)]
  MovingForward -> faceWest [order 2] : [currentHeading == ROB_WEST || currentHeading == ROB_EAST]
  (junction 36) -> SwitchLane [order 2] : [currentHeading == ROB_SOUTH]
      | /moveRequest = MOVE_U_TURN_LEFT;
      | headingRequest = ROB_NORTH;
      | finishCounter = 1;
  (default) -> Idle
  finishZigZag -> Idle : [(currentRoutine == ENU_ZIGZAG)]
  MovingForward -> (junction 33) [order 1] : stopEvent
  (junction 36) -> SwitchLane [order 1] : [currentHeading == ROB_NORTH]
      | /moveRequest = MOVE_U_TURN;
      | headingRequest = ROB_SOUTH;
      | finishCounter++;
  faceWest -> MovingForward : [initHeading]
  Idle -> faceWest : [currentRoutine == ENU_ZIGZAG]
  (junction 33) -> (junction 36) [order 4] : [(sensorView == LEFT_EMPTY_RIGHT_CLEANED)...
      | || (sensorView == LEFT_EMPTY_RIGHT_BUSY)]
  (junction 33) -> (junction 37) [order 3] : [(sensorView == LEFT_BUSY_RIGHT_BUSY)]
  (junction 33) -> (junction 37) [order 5] : [(sensorView == LEFT_BUSY_RIGHT_CLEANED)...
      | || (sensorView == LEFT_CLEANED_RIGHT_BUSY)...
      | || (sensorView == LEFT_CLEANED_RIGHT_CLEANED)]
  SwitchLane -> MovingForward [order 2] : [(headingRequest == currentHeading)...
      | && (targetReached == true)]
  (junction 37) -> SwitchLane [order 1] : [currentHeading == ROB_NORTH]
      | /moveRequest = MOVE_U_TURN;
      | headingRequest = ROB_SOUTH;
      | finishCounter++;
  (junction 37) -> SwitchLane [order 2] : [currentHeading == ROB_SOUTH]
      | /moveRequest = MOVE_U_TURN;
      | headingRequest = ROB_NORTH;
      | finishCounter++;
  data: LEFT_BUSY_RIGHT_EMPTY input; LEFT_CLEANED_RIGHT_EMPTY input; LEFT_EMPTY_RIGHT_BUSY input; LEFT_EMPTY_RIGHT_CLEANED input; LEFT_EMPTY_RIGHT_EMPTY input; LEFT_BUSY_RIGHT_BUSY input; LEFT_CLEANED_RIGHT_CLEANED input; LEFT_BUSY_RIGHT_CLEANED input; LEFT_CLEANED_RIGHT_BUSY input; ROB_NORTH input; ROB_SOUTH input; FORWARD input; MOVE_U_TURN input; MOVE_U_TURN_RIGHT input; MOVE_U_TURN_LEFT input; sensorView input; STOP input; moveRequest output uint8; currentHeading input; currentRoutine input; pumperInterrupt_BOOL input; targetReached input; headingRequest local uint16; ENU_ZIGZAG parameter; zgzgActive output boolean =true;; finishCounter local uint8; CAL_ZgZgCounterThd constant uint8 =CAL_ZgZgCounterThd; initHeading local double; MOVE_TURN_LEFT constant uint8 =ENU_MOVE_TURN_LEFT; MOVE_TURN_RIGHT constant uint8 =ENU_MOVE_TURN_RIGHT; ROB_EAST input =CAL_ROB_EAST; ROB_WEST input =CAL_ROB_WEST
  events: refreshEvent input EITHER_EDGE_EVENT; stopEvent input EITHER_EDGE_EVENT

== stateflow chart RobotControl/StopRoutine/stopRoutine ==
  state stopRoutine
    on every(1,tick):
    send(refreshEvent);
    state hitFinish
      en:
      turnRequest = STOP;
      moveRequest = STOP;
      send(stopEvent);
      hitRoutineRun = false;
    state Run
    state HitStop
      en:
      turnRequest = STOP;
      moveRequest = STOP;
    state backup
      en:
      turnRequest = BACKWARD;
      moveRequest = BACKWARD;
    (default) -> Run
    hitFinish -> Run : [!pumperHit_BOOL]
    Run -> HitStop : [pumperHit_BOOL]
        | /hitRoutineRun = true;
    backup -> hitFinish [order 1] : [i>CAL_backwardTicks]
    HitStop -> backup : [after(10,tick)]/i = 0;
    backup -> (junction 9) [order 2] : [hasChanged(encoderTicks)]
    (junction 9) -> backup : {i++;}
  (default) -> stopRoutine
  data: encoderTicks input; pumperHit_BOOL input; turnRequest output uint8; i local uint8; BACKWARD constant uint8 =ENU_BACKWARD; STOP constant uint8 =ENU_STOP; moveRequest output uint8; hitRoutineRun output boolean; CAL_backwardTicks constant uint8 =CAL_backwardTicks
  events: refreshEvent output EITHER_EDGE_EVENT; stopEvent output EITHER_EDGE_EVENT
